simulink model "BMS_Software"  (R2024b)
settings: configuration reference "BMS_Sw_CodeGenConfig" (kept outside this file)
undefined symbols (not defined in the file): CVM_DMaxVCellMaxCutoff_P, CVM_DMaxVCellMaxDrtd_P, CVM_DMaxVCellMaxWarn_P, CVM_DMaxVCellMinCutoff_P, CVM_DMaxVCellMinDrtd_P, CVM_DMaxVCellMinWarn_P, CVM_DMinVCellMaxCutoff_P, CVM_DMinVCellMaxDrtd_P, CVM_DMinVCellMaxWarn_P, CVM_DMinVCellMinCutoff_P, CVM_DMinVCellMinDrtd_P, CVM_DMinVCellMinWarn_P, CVM_VCellMaxCutoffTh_P, CVM_VCellMaxDrtdTh_P, CVM_VCellMaxWarnTh_P, CVM_VCellMinCutoffTh_P, CVM_VCellMinDrtdTh_P, CVM_VCellMinWarnTh_P, MTM_DMaxTMdulMaxCutoff_P, MTM_DMaxTMdulMaxDrtd_P, MTM_DMaxTMdulMaxWarn_P, MTM_DMaxTMdulMinCutoff_P, MTM_DMaxTMdulMinDrtd_P, MTM_DMaxTMdulMinWarn_P, MTM_DMinTMdulMaxCutoff_P, MTM_DMinTMdulMaxDrtd_P, MTM_DMinTMdulMaxWarn_P, MTM_DMinTMdulMinCutoff_P, MTM_DMinTMdulMinDrtd_P, MTM_DMinTMdulMinWarn_P, MTM_TMdulMaxCutoffTh_P, MTM_TMdulMaxDrtdTh_P, MTM_TMdulMaxWarnTh_P, MTM_TMdulMinCutoffTh_P, MTM_TMdulMinDrtdTh_P, MTM_TMdulMinWarnTh_P, NrCutoff_C, NrDrtd_C, NrNoFlt_C, NrTMdulSnsr_C, NrWarn_C, trun, ts
libraries: BMSLib x12, slrealtimeseriallib x12
settings Model: DataDictionary=BMS_Software_DD.sldd  EnableAccessToBaseWorkspace=off  PauseTimes=0  ExtModeTrigDuration=5  Creator=Chirag Patel  LastModifiedBy=18811
settings ConfigSetRef: SourceName=BMS_Sw_CodeGenConfig

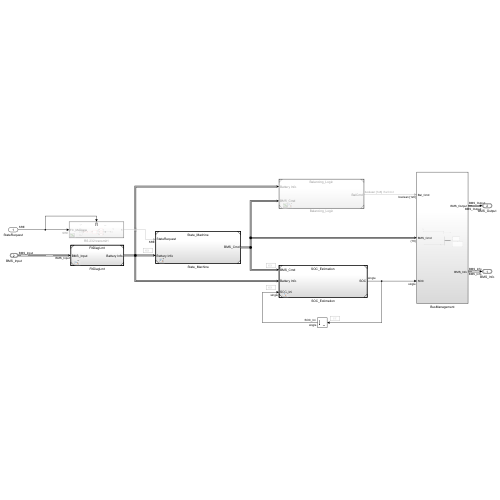
[thumbnail: Simulink's stored preview of the top-level diagram]
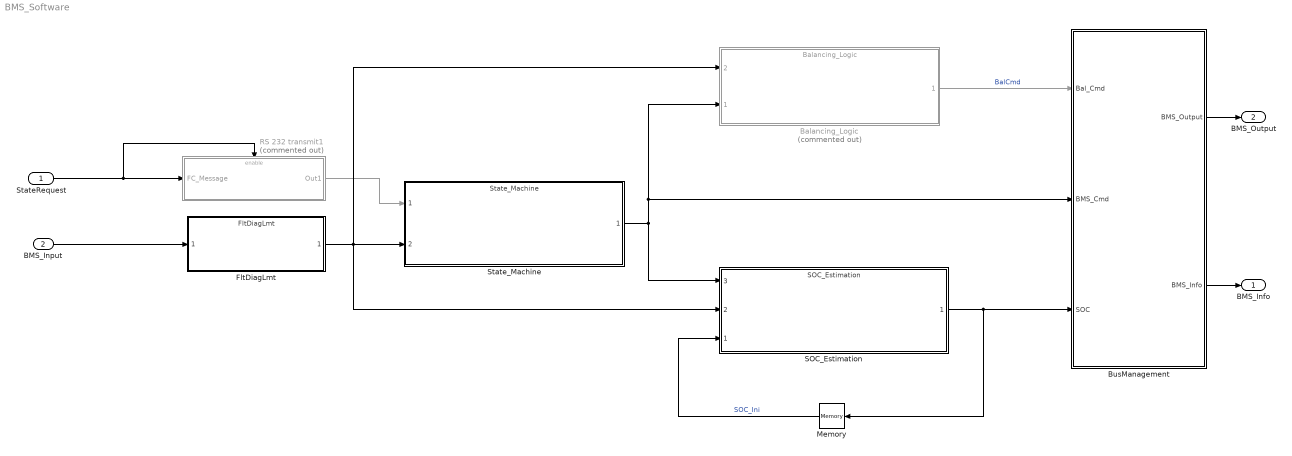
== system BMS_Software ==
  StateRequest : Inport  OutDataTypeStr=Enum: SRE  PortDimensions=1  SampleTime=ts
  BMS_Input : Inport  Port=2  OutDataTypeStr=Bus: BMS_Input  BusOutputAsStruct=on
  Balancing_Logic : ModelReference  Commented=on  ModelNameDialog=Balancing_Logic  SimulationMode=Normal  ModelReferenceVersion=10.5
      settings: PortSchema="{\"entries\":[{\"content\":{\"sides\":[{\"content\":{\"connectorIds\":[\"In2\",\"In1\"]},\"type\":\"ConnectorPlacement.EquallySpacedRectSide\",\"uuid\":\"cc29d713-3759-48d9-a010-cc26194b078c\"},{\"content\":{\"connectorIds\":[\"Out1\"],\"side\":\"RIGHT\"},\"type\":\"ConnectorPlacement.EquallySpacedRectSide\",\"uuid\":\"7e819dab-9dd0-4b9a-8c4e-0d0aaa16d040\"},{\"content\":{\"side\":\"TOP\"},\"type\":\"ConnectorPlacement.EquallySpacedRectSide\",\"uuid\":\"91c10b32-d729-497c-840c-1eed6ab799fc\"}]},\"type\":\"ConnectorPlacement.EquallySpacedConnector\",\"uuid\":\"0865c662-6fe9-4db8-807a-4df99c21aa76\"}],\"packageUris\":[\"http://schema.mathworks.com/mf0/Connector/R2020b\"],\"version\":\"1.0\"}"
  BusManagement : Subsystem
  FltDiagLmt : ModelReference  ModelNameDialog=FltDiagLmt.slx  SimulationMode=Normal  ModelReferenceVersion=10.14
  Memory : Memory
  RS 232 transmit1 : Subsystem  Commented=on
  SOC_Estimation : ModelReference  ModelNameDialog=SOC_Estimation.slx  SimulationMode=Normal  ModelReferenceVersion=10.22
      settings: PortSchema="{\"entries\":[{\"content\":{\"sides\":[{\"content\":{\"connectorIds\":[\"In3\",\"In2\",\"In1\"]},\"type\":\"ConnectorPlacement.EquallySpacedRectSide\",\"uuid\":\"ff68703c-5233-4deb-9e18-bad34cd6bb0f\"},{\"content\":{\"connectorIds\":[\"Out1\"],\"side\":\"RIGHT\"},\"type\":\"ConnectorPlacement.EquallySpacedRectSide\",\"uuid\":\"c5a2e1a1-0f6a-4c93-a24e-98e8f2a93860\"},{\"content\":{\"side\":\"TOP\"},\"type\":\"ConnectorPlacement.EquallySpacedRectSide\",\"uuid\":\"b3729e88-7d1a-421a-a726-893eff6c6b0c\"}]},\"type\":\"ConnectorPlacement.EquallySpacedConnector\",\"uuid\":\"762b3e21-e856-43be-b064-47a21abd58c0\"}],\"packageUris\":[\"http://schema.mathworks.com/mf0/Connector/R2020b\"],\"version\":\"1.0\"}"
  State_Machine : ModelReference  ModelNameDialog=State_Machine  SimulationMode=Normal  ModelReferenceVersion=10.15
  BMS_Info : Outport  OutDataTypeStr=Bus: BMS_Info  VectorParamsAs1DForOutWhenUnconnected=off  BusOutputAsStruct=on
  BMS_Output : Outport  Port=2  OutDataTypeStr=Bus: BMS_Output  VectorParamsAs1DForOutWhenUnconnected=off  BusOutputAsStruct=on
  wires:
  RS 232 transmit1/1(Out1) -> State_Machine/1
  State_Machine/1 -> BusManagement/2(BMS_Cmd), Balancing_Logic/1, SOC_Estimation/3
  BMS_Input/1 -> FltDiagLmt/1
  Memory/1 -> SOC_Estimation/1  "SOC_Ini"
  BusManagement/2(BMS_Info) -> BMS_Info/1
  Balancing_Logic/1 -> BusManagement/1(Bal_Cmd)  "BalCmd"
  FltDiagLmt/1 -> SOC_Estimation/2, Balancing_Logic/2, State_Machine/2
  StateRequest/1 -> RS 232 transmit1/Enable, RS 232 transmit1/1(FC_Message)
  BusManagement/1(BMS_Output) -> BMS_Output/1
  SOC_Estimation/1 -> Memory/1, BusManagement/3(SOC)

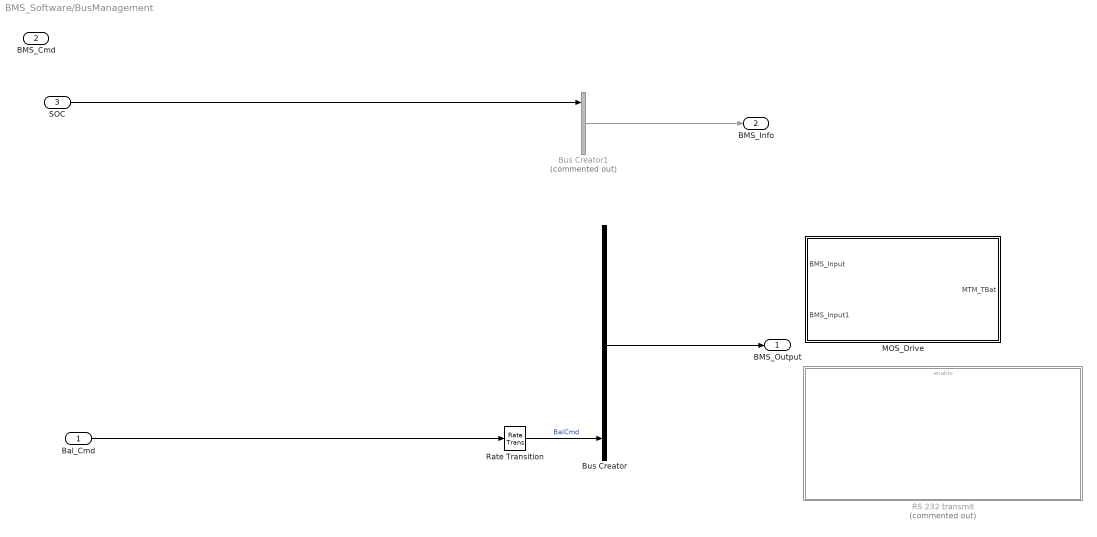
== system BMS_Software/BusManagement ==
  Bal_Cmd : Inport  OutDataTypeStr=boolean
  BMS_Cmd : Inport  Port=2  OutDataTypeStr=Bus: BMS_Cmd
  SOC : Inport  Port=3  OutDataTypeStr=single
  Bus Creator1 : BusCreator  Commented=on  Inputs=3  OutDataTypeStr=Bus: BMS_Info
      settings: InheritFromInputs=off
  Bus Creator : BusCreator  Inputs=10  OutDataTypeStr=Bus: BMS_Output  NonVirtualBus=on
  MOS_Drive : Subsystem
  RS 232 transmit : Subsystem  Commented=on
  Rate Transition : RateTransition  Integrity=off  Deterministic=off
  BMS_Output : Outport
  BMS_Info : Outport  Port=2  OutDataTypeStr=Bus: BMS_Info
  wires:
  Bus Creator1/1 -> BMS_Info/1
  Bus Creator/1 -> BMS_Output/1
  Rate Transition/1 -> Bus Creator/10  "BalCmd"
  Bal_Cmd/1 -> Rate Transition/1
  SOC/1 -> Bus Creator1/1

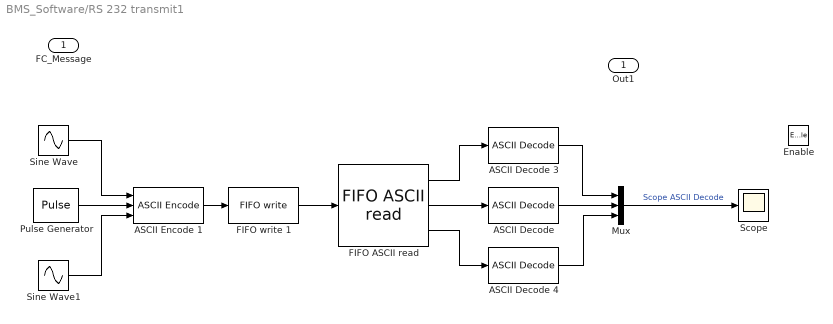
== system BMS_Software/RS 232 transmit1 ==
  FC_Message : Inport  OutDataTypeStr=Enum: SRE  PortDimensions=1  SampleTime=ts
  Enable : EnablePort
  "ASCII Decode " : slrealtimeseriallib/ASCII Decode  format=pulse %d\r\n  nvars=1  vartypes={ }
  ASCII Decode 3 : slrealtimeseriallib/ASCII Decode  format=sine1 %f\r\n  nvars=1  vartypes={ }
  ASCII Decode 4 : slrealtimeseriallib/ASCII Decode  format=sine2 %f\r\n  nvars=1  vartypes={ }
  ASCII Encode 1 : slrealtimeseriallib/ASCII Encode  format=foo sine1 %f\r\n bar pulse %d\r\n fud sine2 %f\r\n  nvars=3  maxlength=128  vartypes={ 'double' }
  "FIFO ASCII read " : slrealtimeseriallib/FIFO ASCII read  header={'sine1','pulse','sine2'}  term=[13 10]  hold=Zero output if no new data  enable=off  maxsize=1024  outputtype=8 bit uint null terminated  sampletime=trun
  FIFO write 1 : slrealtimeseriallib/FIFO write  size=1024  inputtype=8 bit uint null terminated  present=off  sampletime=trun
  Mux : Mux  Inputs=3
  Pulse Generator : DiscretePulseGenerator  Period=101  PulseWidth=50  SampleTime=trun
  Scope : Scope
  Sine Wave : Sin  Amplitude=2  Bias=1  Frequency=10.1  SampleTime=trun
  Sine Wave1 : Sin  Bias=-1  Frequency=10.11  Phase=3.14  SampleTime=trun
  Out1 : Outport
  wires:
  FIFO write 1/1 -> "FIFO ASCII read "/1
  "FIFO ASCII read "/3 -> ASCII Decode 4/1
  Sine Wave/1 -> ASCII Encode 1/1
  Mux/1 -> Scope/1  "Scope ASCII Decode"
  Pulse Generator/1 -> ASCII Encode 1/2
  "ASCII Decode "/1 -> Mux/2
  ASCII Encode 1/1 -> FIFO write 1/1
  ASCII Decode 4/1 -> Mux/3
  ASCII Decode 3/1 -> Mux/1
  "FIFO ASCII read "/2 -> "ASCII Decode "/1
  "FIFO ASCII read "/1 -> ASCII Decode 3/1
  Sine Wave1/1 -> ASCII Encode 1/3

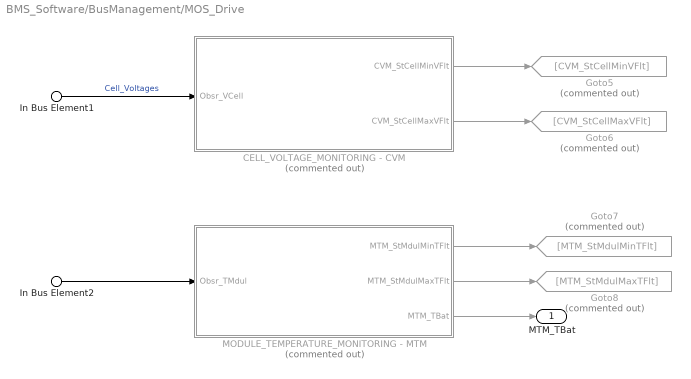
== system BMS_Software/BusManagement/MOS_Drive ==
  In Bus Element1 : Inport  PortName=BMS_Input  Element=Cell_Voltages
  In Bus Element2 : Inport  Port=2  PortName=BMS_Input1  Element=Cell_Temperatures
  CELL_VOLTAGE_MONITORING - CVM : Subsystem  Commented=on
  Goto5 : Goto  Commented=on  GotoTag=CVM_StCellMinVFlt
  Goto6 : Goto  Commented=on  GotoTag=CVM_StCellMaxVFlt
  Goto7 : Goto  Commented=on  GotoTag=MTM_StMdulMinTFlt
  Goto8 : Goto  Commented=on  GotoTag=MTM_StMdulMaxTFlt
  MODULE_TEMPERATURE_MONITORING - MTM : Subsystem  Commented=on
  MTM_TBat : Outport  VectorParamsAs1DForOutWhenUnconnected=off
  wires:
  CELL_VOLTAGE_MONITORING - CVM/2(CVM_StCellMaxVFlt) -> Goto6/1
  CELL_VOLTAGE_MONITORING - CVM/1(CVM_StCellMinVFlt) -> Goto5/1
  In Bus Element1/1 -> CELL_VOLTAGE_MONITORING - CVM/1(Obsr_VCell)  "Cell_Voltages"
  MODULE_TEMPERATURE_MONITORING - MTM/3(MTM_TBat) -> MTM_TBat/1
  MODULE_TEMPERATURE_MONITORING - MTM/1(MTM_StMdulMinTFlt) -> Goto7/1
  MODULE_TEMPERATURE_MONITORING - MTM/2(MTM_StMdulMaxTFlt) -> Goto8/1
  In Bus Element2/1 -> MODULE_TEMPERATURE_MONITORING - MTM/1(Obsr_TMdul)

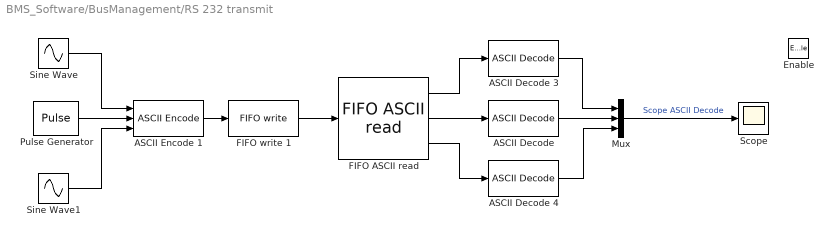
== system BMS_Software/BusManagement/RS 232 transmit ==
  Enable : EnablePort
  "ASCII Decode " : slrealtimeseriallib/ASCII Decode  format=pulse %d\r\n  nvars=1  vartypes={ }
  ASCII Decode 3 : slrealtimeseriallib/ASCII Decode  format=sine1 %f\r\n  nvars=1  vartypes={ }
  ASCII Decode 4 : slrealtimeseriallib/ASCII Decode  format=sine2 %f\r\n  nvars=1  vartypes={ }
  ASCII Encode 1 : slrealtimeseriallib/ASCII Encode  format=foo sine1 %f\r\n bar pulse %d\r\n fud sine2 %f\r\n  nvars=3  maxlength=128  vartypes={ 'double' }
  "FIFO ASCII read " : slrealtimeseriallib/FIFO ASCII read  header={'sine1','pulse','sine2'}  term=[13 10]  hold=Zero output if no new data  enable=off  maxsize=1024  outputtype=8 bit uint null terminated  sampletime=trun
  FIFO write 1 : slrealtimeseriallib/FIFO write  size=1024  inputtype=8 bit uint null terminated  present=off  sampletime=trun
  Mux : Mux  Inputs=3
  Pulse Generator : DiscretePulseGenerator  Period=101  PulseWidth=50  SampleTime=trun
  Scope : Scope
  Sine Wave : Sin  Amplitude=2  Bias=1  Frequency=10.1  SampleTime=trun
  Sine Wave1 : Sin  Bias=-1  Frequency=10.11  Phase=3.14  SampleTime=trun
  wires:
  FIFO write 1/1 -> "FIFO ASCII read "/1
  "FIFO ASCII read "/3 -> ASCII Decode 4/1
  Sine Wave/1 -> ASCII Encode 1/1
  Mux/1 -> Scope/1  "Scope ASCII Decode"
  Pulse Generator/1 -> ASCII Encode 1/2
  "ASCII Decode "/1 -> Mux/2
  ASCII Encode 1/1 -> FIFO write 1/1
  ASCII Decode 4/1 -> Mux/3
  ASCII Decode 3/1 -> Mux/1
  "FIFO ASCII read "/2 -> "ASCII Decode "/1
  "FIFO ASCII read "/1 -> ASCII Decode 3/1
  Sine Wave1/1 -> ASCII Encode 1/3

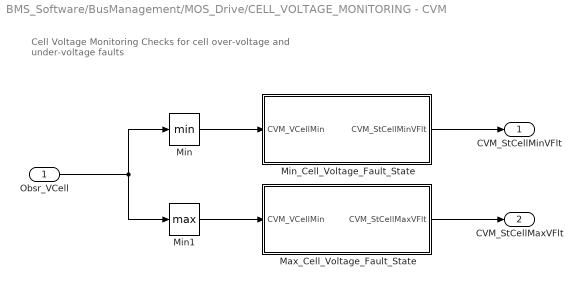
== system BMS_Software/BusManagement/MOS_Drive/CELL_VOLTAGE_MONITORING - CVM ==
  note: Cell Voltage Monitoring
      |
      | Checks for cell over-voltage and under-voltage faults
  Obsr_VCell : Inport
  Max_Cell_Voltage_Fault_State : Subsystem
  Min : MinMax
  Min1 : MinMax  Function=max
  Min_Cell_Voltage_Fault_State : Subsystem
  CVM_StCellMinVFlt : Outport  VectorParamsAs1DForOutWhenUnconnected=off
  CVM_StCellMaxVFlt : Outport  Port=2  VectorParamsAs1DForOutWhenUnconnected=off
  wires:
  Obsr_VCell/1 -> Min/1, Min1/1
  Min/1 -> Min_Cell_Voltage_Fault_State/1(CVM_VCellMin)
  Min1/1 -> Max_Cell_Voltage_Fault_State/1(CVM_VCellMin)
  Min_Cell_Voltage_Fault_State/1(CVM_StCellMinVFlt) -> CVM_StCellMinVFlt/1
  Max_Cell_Voltage_Fault_State/1(CVM_StCellMaxVFlt) -> CVM_StCellMaxVFlt/1

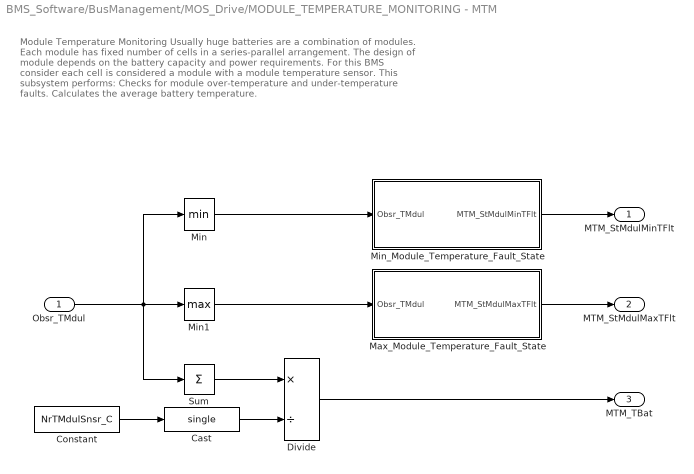
== system BMS_Software/BusManagement/MOS_Drive/MODULE_TEMPERATURE_MONITORING - MTM ==
  note: Module Temperature Monitoring
      |
      | Usually huge batteries are a combination of modules. Each module has fixed number of cells in a series-parallel arrangement. The design of module depends on the battery capacity and power requirements. For this BMS consider each cell is considered a module with a module temperature sensor. This subsystem performs:
      |
      | Checks for module over-temperature and under-temperature faults.
      |
      | Calculates the average battery temperature.
  Obsr_TMdul : Inport
  Cast : DataTypeConversion  OutDataTypeStr=single  SaturateOnIntegerOverflow=off  RndMeth=Floor
  Constant : Constant  Value=NrTMdulSnsr_C
  Divide : Product  Inputs=*/
  Max_Module_Temperature_Fault_State : Subsystem
  Min : MinMax
  Min1 : MinMax  Function=max
  Min_Module_Temperature_Fault_State : Subsystem
  Sum : Sum  Inputs=+
  MTM_StMdulMinTFlt : Outport  VectorParamsAs1DForOutWhenUnconnected=off
  MTM_StMdulMaxTFlt : Outport  Port=2  VectorParamsAs1DForOutWhenUnconnected=off
  MTM_TBat : Outport  Port=3  VectorParamsAs1DForOutWhenUnconnected=off
  wires:
  Min1/1 -> Max_Module_Temperature_Fault_State/1(Obsr_TMdul)
  Max_Module_Temperature_Fault_State/1(MTM_StMdulMaxTFlt) -> MTM_StMdulMaxTFlt/1
  Min/1 -> Min_Module_Temperature_Fault_State/1(Obsr_TMdul)
  Min_Module_Temperature_Fault_State/1(MTM_StMdulMinTFlt) -> MTM_StMdulMinTFlt/1
  Obsr_TMdul/1 -> Min/1, Sum/1, Min1/1
  Sum/1 -> Divide/1
  Divide/1 -> MTM_TBat/1
  Constant/1 -> Cast/1
  Cast/1 -> Divide/2

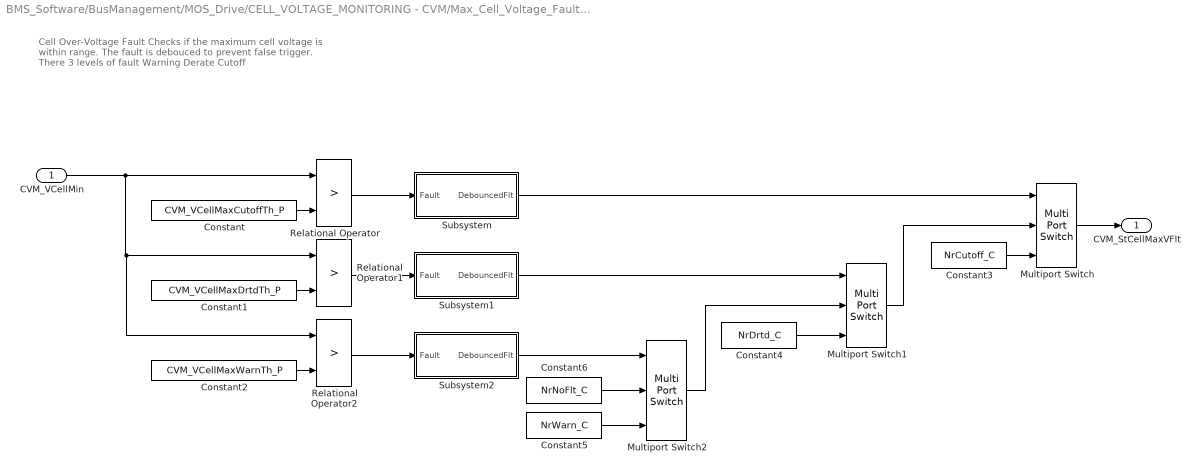
== system BMS_Software/BusManagement/MOS_Drive/CELL_VOLTAGE_MONITORING - CVM/Max_Cell_Voltage_Fault_State ==
  note: Cell Over-Voltage Fault
      |
      | Checks if the maximum cell voltage is within range. The fault is debouced to prevent false trigger.
      |
      | There 3 levels of fault
      | Warning
      | Derate
      | Cutoff
  CVM_VCellMin : Inport
  Constant : Constant  Value=CVM_VCellMaxCutoffTh_P
  Constant1 : Constant  Value=CVM_VCellMaxDrtdTh_P
  Constant2 : Constant  Value=CVM_VCellMaxWarnTh_P
  Constant3 : Constant  Value=NrCutoff_C
  Constant4 : Constant  Value=NrDrtd_C
  Constant5 : Constant  Value=NrWarn_C
  Constant6 : Constant  Value=NrNoFlt_C
  Multiport Switch : MultiPortSwitch  DataPortOrder=Zero-based contiguous  Inputs=2  zeroidx=on  SaturateOnIntegerOverflow=off  InputSameDT=off
  Multiport Switch1 : MultiPortSwitch  DataPortOrder=Zero-based contiguous  Inputs=2  zeroidx=on  SaturateOnIntegerOverflow=off  InputSameDT=off
  Multiport Switch2 : MultiPortSwitch  DataPortOrder=Zero-based contiguous  Inputs=2  zeroidx=on  SaturateOnIntegerOverflow=off  InputSameDT=off
  Relational Operator : RelationalOperator  Operator=>  OutDataTypeStr=boolean  RndMeth=Simplest  InputSameDT=off
  Relational Operator1 : RelationalOperator  Operator=>  OutDataTypeStr=boolean  RndMeth=Simplest  InputSameDT=off
  Relational Operator2 : RelationalOperator  Operator=>  OutDataTypeStr=boolean  RndMeth=Simplest  InputSameDT=off
  Subsystem : Subsystem
  Subsystem1 : Subsystem
  Subsystem2 : Subsystem
  CVM_StCellMaxVFlt : Outport  VectorParamsAs1DForOutWhenUnconnected=off
  wires:
  Constant6/1 -> Multiport Switch2/2
  Constant5/1 -> Multiport Switch2/3
  Constant2/1 -> Relational Operator2/2
  Multiport Switch2/1 -> Multiport Switch1/2
  Constant4/1 -> Multiport Switch1/3
  Constant1/1 -> Relational Operator1/2
  Constant3/1 -> Multiport Switch/3
  Multiport Switch1/1 -> Multiport Switch/2
  Constant/1 -> Relational Operator/2
  Multiport Switch/1 -> CVM_StCellMaxVFlt/1
  CVM_VCellMin/1 -> Relational Operator/1, Relational Operator1/1, Relational Operator2/1
  Relational Operator2/1 -> Subsystem2/1(Fault)
  Subsystem/1(DebouncedFlt) -> Multiport Switch/1
  Relational Operator/1 -> Subsystem/1(Fault)
  Relational Operator1/1 -> Subsystem1/1(Fault)
  Subsystem1/1(DebouncedFlt) -> Multiport Switch1/1
  Subsystem2/1(DebouncedFlt) -> Multiport Switch2/1

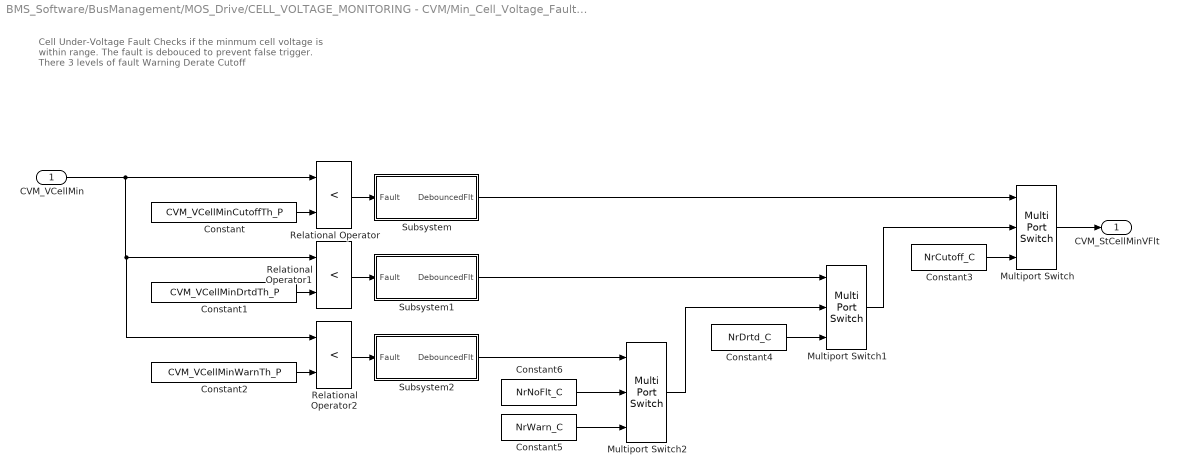
== system BMS_Software/BusManagement/MOS_Drive/CELL_VOLTAGE_MONITORING - CVM/Min_Cell_Voltage_Fault_State ==
  note: Cell Under-Voltage Fault
      |
      | Checks if the minmum cell voltage is within range. The fault is debouced to prevent false trigger.
      |
      | There 3 levels of fault
      | Warning
      | Derate
      | Cutoff
  CVM_VCellMin : Inport
  Constant : Constant  Value=CVM_VCellMinCutoffTh_P
  Constant1 : Constant  Value=CVM_VCellMinDrtdTh_P
  Constant2 : Constant  Value=CVM_VCellMinWarnTh_P
  Constant3 : Constant  Value=NrCutoff_C
  Constant4 : Constant  Value=NrDrtd_C
  Constant5 : Constant  Value=NrWarn_C
  Constant6 : Constant  Value=NrNoFlt_C
  Multiport Switch : MultiPortSwitch  DataPortOrder=Zero-based contiguous  Inputs=2  zeroidx=on  SaturateOnIntegerOverflow=off  InputSameDT=off
  Multiport Switch1 : MultiPortSwitch  DataPortOrder=Zero-based contiguous  Inputs=2  zeroidx=on  SaturateOnIntegerOverflow=off  InputSameDT=off
  Multiport Switch2 : MultiPortSwitch  DataPortOrder=Zero-based contiguous  Inputs=2  zeroidx=on  SaturateOnIntegerOverflow=off  InputSameDT=off
  Relational Operator : RelationalOperator  Operator=<  OutDataTypeStr=boolean  RndMeth=Simplest  InputSameDT=off
  Relational Operator1 : RelationalOperator  Operator=<  OutDataTypeStr=boolean  RndMeth=Simplest  InputSameDT=off
  Relational Operator2 : RelationalOperator  Operator=<  OutDataTypeStr=boolean  RndMeth=Simplest  InputSameDT=off
  Subsystem : Subsystem
  Subsystem1 : Subsystem
  Subsystem2 : Subsystem
  CVM_StCellMinVFlt : Outport  VectorParamsAs1DForOutWhenUnconnected=off
  wires:
  CVM_VCellMin/1 -> Relational Operator2/1, Relational Operator1/1, Relational Operator/1
  Multiport Switch/1 -> CVM_StCellMinVFlt/1
  Relational Operator/1 -> Subsystem/1(Fault)
  Constant/1 -> Relational Operator/2
  Multiport Switch1/1 -> Multiport Switch/2
  Constant3/1 -> Multiport Switch/3
  Relational Operator1/1 -> Subsystem1/1(Fault)
  Constant1/1 -> Relational Operator1/2
  Constant4/1 -> Multiport Switch1/3
  Multiport Switch2/1 -> Multiport Switch1/2
  Relational Operator2/1 -> Subsystem2/1(Fault)
  Constant2/1 -> Relational Operator2/2
  Constant5/1 -> Multiport Switch2/3
  Constant6/1 -> Multiport Switch2/2
  Subsystem/1(DebouncedFlt) -> Multiport Switch/1
  Subsystem1/1(DebouncedFlt) -> Multiport Switch1/1
  Subsystem2/1(DebouncedFlt) -> Multiport Switch2/1

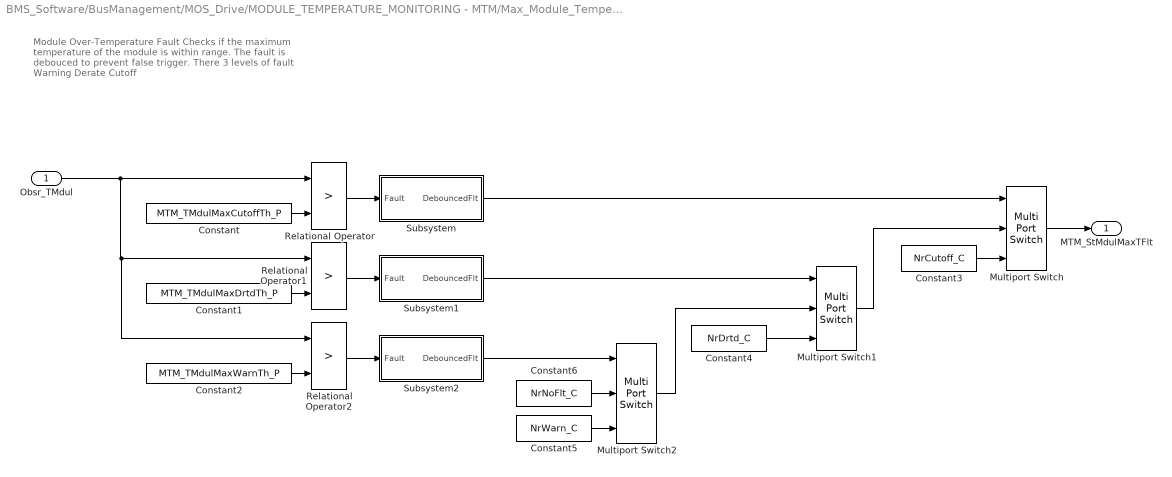
== system BMS_Software/BusManagement/MOS_Drive/MODULE_TEMPERATURE_MONITORING - MTM/Max_Module_Temperature_Fault_State ==
  note: Module Over-Temperature Fault
      |
      | Checks if the maximum temperature of the module is within range. The fault is debouced to prevent false trigger.
      |
      | There 3 levels of fault
      | Warning
      | Derate
      | Cutoff
  Obsr_TMdul : Inport
  Constant : Constant  Value=MTM_TMdulMaxCutoffTh_P
  Constant1 : Constant  Value=MTM_TMdulMaxDrtdTh_P
  Constant2 : Constant  Value=MTM_TMdulMaxWarnTh_P
  Constant3 : Constant  Value=NrCutoff_C
  Constant4 : Constant  Value=NrDrtd_C
  Constant5 : Constant  Value=NrWarn_C
  Constant6 : Constant  Value=NrNoFlt_C
  Multiport Switch : MultiPortSwitch  DataPortOrder=Zero-based contiguous  Inputs=2  zeroidx=on  SaturateOnIntegerOverflow=off  InputSameDT=off
  Multiport Switch1 : MultiPortSwitch  DataPortOrder=Zero-based contiguous  Inputs=2  zeroidx=on  SaturateOnIntegerOverflow=off  InputSameDT=off
  Multiport Switch2 : MultiPortSwitch  DataPortOrder=Zero-based contiguous  Inputs=2  zeroidx=on  SaturateOnIntegerOverflow=off  InputSameDT=off
  Relational Operator : RelationalOperator  Operator=>  OutDataTypeStr=boolean  RndMeth=Simplest  InputSameDT=off
  Relational Operator1 : RelationalOperator  Operator=>  OutDataTypeStr=boolean  RndMeth=Simplest  InputSameDT=off
  Relational Operator2 : RelationalOperator  Operator=>  OutDataTypeStr=boolean  RndMeth=Simplest  InputSameDT=off
  Subsystem : Subsystem
  Subsystem1 : Subsystem
  Subsystem2 : Subsystem
  MTM_StMdulMaxTFlt : Outport  VectorParamsAs1DForOutWhenUnconnected=off
  wires:
  Constant6/1 -> Multiport Switch2/2
  Constant5/1 -> Multiport Switch2/3
  Constant2/1 -> Relational Operator2/2
  Relational Operator2/1 -> Subsystem2/1(Fault)
  Multiport Switch2/1 -> Multiport Switch1/2
  Constant4/1 -> Multiport Switch1/3
  Constant1/1 -> Relational Operator1/2
  Relational Operator1/1 -> Subsystem1/1(Fault)
  Constant3/1 -> Multiport Switch/3
  Multiport Switch1/1 -> Multiport Switch/2
  Constant/1 -> Relational Operator/2
  Relational Operator/1 -> Subsystem/1(Fault)
  Multiport Switch/1 -> MTM_StMdulMaxTFlt/1
  Obsr_TMdul/1 -> Relational Operator/1, Relational Operator1/1, Relational Operator2/1
  Subsystem/1(DebouncedFlt) -> Multiport Switch/1
  Subsystem1/1(DebouncedFlt) -> Multiport Switch1/1
  Subsystem2/1(DebouncedFlt) -> Multiport Switch2/1

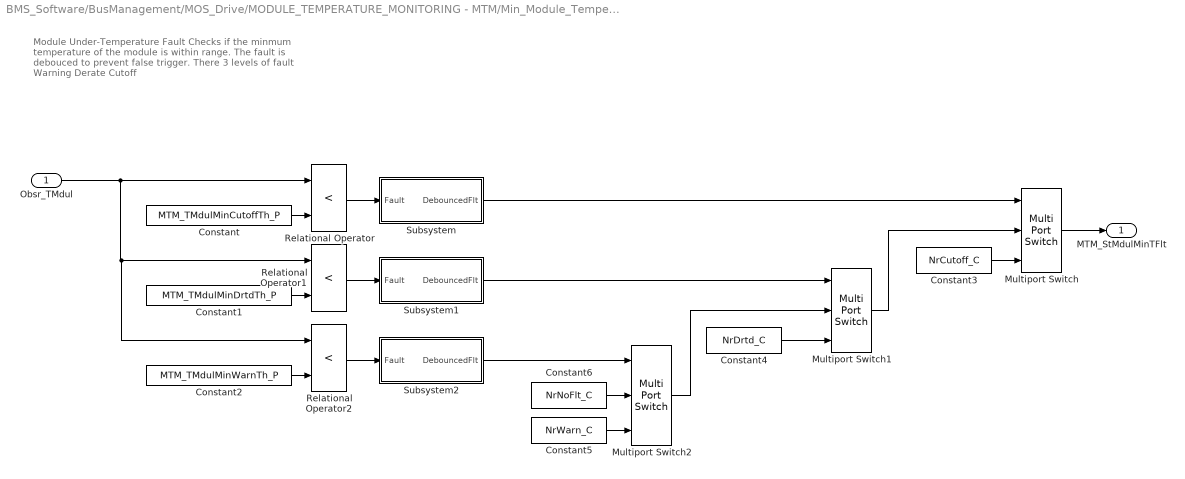
== system BMS_Software/BusManagement/MOS_Drive/MODULE_TEMPERATURE_MONITORING - MTM/Min_Module_Temperature_Fault_State ==
  note: Module Under-Temperature Fault
      |
      | Checks if the minmum temperature of the module is within range. The fault is debouced to prevent false trigger.
      |
      | There 3 levels of fault
      | Warning
      | Derate
      | Cutoff
  Obsr_TMdul : Inport
  Constant : Constant  Value=MTM_TMdulMinCutoffTh_P
  Constant1 : Constant  Value=MTM_TMdulMinDrtdTh_P
  Constant2 : Constant  Value=MTM_TMdulMinWarnTh_P
  Constant3 : Constant  Value=NrCutoff_C
  Constant4 : Constant  Value=NrDrtd_C
  Constant5 : Constant  Value=NrWarn_C
  Constant6 : Constant  Value=NrNoFlt_C
  Multiport Switch : MultiPortSwitch  DataPortOrder=Zero-based contiguous  Inputs=2  zeroidx=on  SaturateOnIntegerOverflow=off  InputSameDT=off
  Multiport Switch1 : MultiPortSwitch  DataPortOrder=Zero-based contiguous  Inputs=2  zeroidx=on  SaturateOnIntegerOverflow=off  InputSameDT=off
  Multiport Switch2 : MultiPortSwitch  DataPortOrder=Zero-based contiguous  Inputs=2  zeroidx=on  SaturateOnIntegerOverflow=off  InputSameDT=off
  Relational Operator : RelationalOperator  Operator=<  OutDataTypeStr=boolean  RndMeth=Simplest  InputSameDT=off
  Relational Operator1 : RelationalOperator  Operator=<  OutDataTypeStr=boolean  RndMeth=Simplest  InputSameDT=off
  Relational Operator2 : RelationalOperator  Operator=<  OutDataTypeStr=boolean  RndMeth=Simplest  InputSameDT=off
  Subsystem : Subsystem
  Subsystem1 : Subsystem
  Subsystem2 : Subsystem
  MTM_StMdulMinTFlt : Outport  VectorParamsAs1DForOutWhenUnconnected=off
  wires:
  Obsr_TMdul/1 -> Relational Operator2/1, Relational Operator1/1, Relational Operator/1
  Multiport Switch/1 -> MTM_StMdulMinTFlt/1
  Relational Operator/1 -> Subsystem/1(Fault)
  Constant/1 -> Relational Operator/2
  Multiport Switch1/1 -> Multiport Switch/2
  Constant3/1 -> Multiport Switch/3
  Relational Operator1/1 -> Subsystem1/1(Fault)
  Constant1/1 -> Relational Operator1/2
  Constant4/1 -> Multiport Switch1/3
  Multiport Switch2/1 -> Multiport Switch1/2
  Relational Operator2/1 -> Subsystem2/1(Fault)
  Constant2/1 -> Relational Operator2/2
  Constant5/1 -> Multiport Switch2/3
  Constant6/1 -> Multiport Switch2/2
  Subsystem/1(DebouncedFlt) -> Multiport Switch/1
  Subsystem1/1(DebouncedFlt) -> Multiport Switch1/1
  Subsystem2/1(DebouncedFlt) -> Multiport Switch2/1

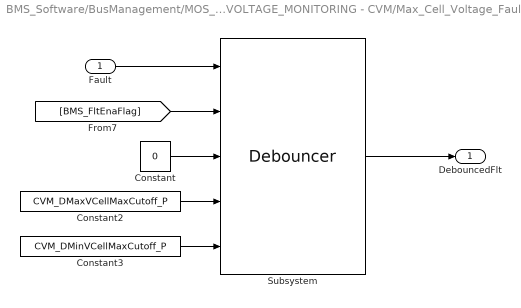
== system BMS_Software/BusManagement/MOS_Drive/CELL_VOLTAGE_MONITORING - CVM/Max_Cell_Voltage_Fault_State/Subsystem ==
  Fault : Inport
  Constant : Constant  Value=0
  Constant2 : Constant  Value=CVM_DMaxVCellMaxCutoff_P
  Constant3 : Constant  Value=CVM_DMinVCellMaxCutoff_P
  Subsystem : BMSLib/Debouncer
  DebouncedFlt : Outport  VectorParamsAs1DForOutWhenUnconnected=off
  wires:
  Fault/1 -> Subsystem/1
  Subsystem/1 -> DebouncedFlt/1
  [BMS_FltEnaFlag] -> Subsystem/2
  Constant/1 -> Subsystem/3
  Constant2/1 -> Subsystem/4
  Constant3/1 -> Subsystem/5

== system BMS_Software/BusManagement/MOS_Drive/CELL_VOLTAGE_MONITORING - CVM/Max_Cell_Voltage_Fault_State/Subsystem1 ==
  Fault : Inport
  Constant1 : Constant  Value=0
  Constant2 : Constant  Value=CVM_DMaxVCellMaxDrtd_P
  Constant3 : Constant  Value=CVM_DMinVCellMaxDrtd_P
  Subsystem : BMSLib/Debouncer
  DebouncedFlt : Outport  VectorParamsAs1DForOutWhenUnconnected=off
  wires:
  Constant3/1 -> Subsystem/5
  Constant2/1 -> Subsystem/4
  Constant1/1 -> Subsystem/3
  [BMS_FltEnaFlag] -> Subsystem/2
  Subsystem/1 -> DebouncedFlt/1
  Fault/1 -> Subsystem/1

== system BMS_Software/BusManagement/MOS_Drive/CELL_VOLTAGE_MONITORING - CVM/Max_Cell_Voltage_Fault_State/Subsystem2 ==
  Fault : Inport
  Constant1 : Constant  Value=0
  Constant2 : Constant  Value=CVM_DMaxVCellMaxWarn_P
  Constant3 : Constant  Value=CVM_DMinVCellMaxWarn_P
  Subsystem : BMSLib/Debouncer
  DebouncedFlt : Outport  VectorParamsAs1DForOutWhenUnconnected=off
  wires:
  Fault/1 -> Subsystem/1
  Subsystem/1 -> DebouncedFlt/1
  [BMS_FltEnaFlag] -> Subsystem/2
  Constant1/1 -> Subsystem/3
  Constant2/1 -> Subsystem/4
  Constant3/1 -> Subsystem/5

== system BMS_Software/BusManagement/MOS_Drive/CELL_VOLTAGE_MONITORING - CVM/Min_Cell_Voltage_Fault_State/Subsystem ==
  Fault : Inport
  Constant1 : Constant  Value=0
  Constant2 : Constant  Value=CVM_DMaxVCellMinCutoff_P
  Constant3 : Constant  Value=CVM_DMinVCellMinCutoff_P
  Subsystem : BMSLib/Debouncer
  DebouncedFlt : Outport  VectorParamsAs1DForOutWhenUnconnected=off
  wires:
  Fault/1 -> Subsystem/1
  Subsystem/1 -> DebouncedFlt/1
  [BMS_FltEnaFlag] -> Subsystem/2
  Constant1/1 -> Subsystem/3
  Constant2/1 -> Subsystem/4
  Constant3/1 -> Subsystem/5

== system BMS_Software/BusManagement/MOS_Drive/CELL_VOLTAGE_MONITORING - CVM/Min_Cell_Voltage_Fault_State/Subsystem1 ==
  Fault : Inport
  Constant1 : Constant  Value=0
  Constant2 : Constant  Value=CVM_DMaxVCellMinDrtd_P
  Constant3 : Constant  Value=CVM_DMinVCellMinDrtd_P
  Subsystem : BMSLib/Debouncer
  DebouncedFlt : Outport  VectorParamsAs1DForOutWhenUnconnected=off
  wires:
  Constant3/1 -> Subsystem/5
  Constant2/1 -> Subsystem/4
  Constant1/1 -> Subsystem/3
  [BMS_FltEnaFlag] -> Subsystem/2
  Subsystem/1 -> DebouncedFlt/1
  Fault/1 -> Subsystem/1

== system BMS_Software/BusManagement/MOS_Drive/CELL_VOLTAGE_MONITORING - CVM/Min_Cell_Voltage_Fault_State/Subsystem2 ==
  Fault : Inport
  Constant1 : Constant  Value=0
  Constant2 : Constant  Value=CVM_DMaxVCellMinWarn_P
  Constant3 : Constant  Value=CVM_DMinVCellMinWarn_P
  Subsystem : BMSLib/Debouncer
  DebouncedFlt : Outport  VectorParamsAs1DForOutWhenUnconnected=off
  wires:
  Fault/1 -> Subsystem/1
  Subsystem/1 -> DebouncedFlt/1
  [BMS_FltEnaFlag] -> Subsystem/2
  Constant1/1 -> Subsystem/3
  Constant2/1 -> Subsystem/4
  Constant3/1 -> Subsystem/5

== system BMS_Software/BusManagement/MOS_Drive/MODULE_TEMPERATURE_MONITORING - MTM/Max_Module_Temperature_Fault_State/Subsystem ==
  Fault : Inport
  Constant1 : Constant  Value=0
  Constant2 : Constant  Value=MTM_DMaxTMdulMaxCutoff_P
  Constant3 : Constant  Value=MTM_DMinTMdulMaxCutoff_P
  Subsystem : BMSLib/Debouncer
  DebouncedFlt : Outport  VectorParamsAs1DForOutWhenUnconnected=off
  wires:
  Fault/1 -> Subsystem/1
  Subsystem/1 -> DebouncedFlt/1
  [BMS_FltEnaFlag] -> Subsystem/2
  Constant1/1 -> Subsystem/3
  Constant2/1 -> Subsystem/4
  Constant3/1 -> Subsystem/5

== system BMS_Software/BusManagement/MOS_Drive/MODULE_TEMPERATURE_MONITORING - MTM/Max_Module_Temperature_Fault_State/Subsystem1 ==
  Fault : Inport
  Constant1 : Constant  Value=0
  Constant2 : Constant  Value=MTM_DMaxTMdulMaxDrtd_P
  Constant3 : Constant  Value=MTM_DMinTMdulMaxDrtd_P
  Subsystem : BMSLib/Debouncer
  DebouncedFlt : Outport  VectorParamsAs1DForOutWhenUnconnected=off
  wires:
  Constant3/1 -> Subsystem/5
  Constant2/1 -> Subsystem/4
  Constant1/1 -> Subsystem/3
  [BMS_FltEnaFlag] -> Subsystem/2
  Subsystem/1 -> DebouncedFlt/1
  Fault/1 -> Subsystem/1

== system BMS_Software/BusManagement/MOS_Drive/MODULE_TEMPERATURE_MONITORING - MTM/Max_Module_Temperature_Fault_State/Subsystem2 ==
  Fault : Inport
  Constant1 : Constant  Value=0
  Constant2 : Constant  Value=MTM_DMaxTMdulMaxWarn_P
  Constant3 : Constant  Value=MTM_DMinTMdulMaxWarn_P
  Subsystem : BMSLib/Debouncer
  DebouncedFlt : Outport  VectorParamsAs1DForOutWhenUnconnected=off
  wires:
  Fault/1 -> Subsystem/1
  Subsystem/1 -> DebouncedFlt/1
  [BMS_FltEnaFlag] -> Subsystem/2
  Constant1/1 -> Subsystem/3
  Constant2/1 -> Subsystem/4
  Constant3/1 -> Subsystem/5

== system BMS_Software/BusManagement/MOS_Drive/MODULE_TEMPERATURE_MONITORING - MTM/Min_Module_Temperature_Fault_State/Subsystem ==
  Fault : Inport
  Constant1 : Constant  Value=0
  Constant2 : Constant  Value=MTM_DMaxTMdulMinCutoff_P
  Constant3 : Constant  Value=MTM_DMinTMdulMinCutoff_P
  Subsystem : BMSLib/Debouncer
  DebouncedFlt : Outport  VectorParamsAs1DForOutWhenUnconnected=off
  wires:
  Fault/1 -> Subsystem/1
  Subsystem/1 -> DebouncedFlt/1
  [BMS_FltEnaFlag] -> Subsystem/2
  Constant1/1 -> Subsystem/3
  Constant2/1 -> Subsystem/4
  Constant3/1 -> Subsystem/5

== system BMS_Software/BusManagement/MOS_Drive/MODULE_TEMPERATURE_MONITORING - MTM/Min_Module_Temperature_Fault_State/Subsystem1 ==
  Fault : Inport
  Constant1 : Constant  Value=0
  Constant2 : Constant  Value=MTM_DMaxTMdulMinDrtd_P
  Constant3 : Constant  Value=MTM_DMinTMdulMinDrtd_P
  Subsystem : BMSLib/Debouncer
  DebouncedFlt : Outport  VectorParamsAs1DForOutWhenUnconnected=off
  wires:
  Constant3/1 -> Subsystem/5
  Constant2/1 -> Subsystem/4
  Constant1/1 -> Subsystem/3
  [BMS_FltEnaFlag] -> Subsystem/2
  Subsystem/1 -> DebouncedFlt/1
  Fault/1 -> Subsystem/1

== system BMS_Software/BusManagement/MOS_Drive/MODULE_TEMPERATURE_MONITORING - MTM/Min_Module_Temperature_Fault_State/Subsystem2 ==
  Fault : Inport
  Constant1 : Constant  Value=0
  Constant2 : Constant  Value=MTM_DMaxTMdulMinWarn_P
  Constant3 : Constant  Value=MTM_DMinTMdulMinWarn_P
  Subsystem : BMSLib/Debouncer
  DebouncedFlt : Outport  VectorParamsAs1DForOutWhenUnconnected=off
  wires:
  Fault/1 -> Subsystem/1
  Subsystem/1 -> DebouncedFlt/1
  [BMS_FltEnaFlag] -> Subsystem/2
  Constant1/1 -> Subsystem/3
  Constant2/1 -> Subsystem/4
  Constant3/1 -> Subsystem/5
